simulink model "weightedSystem"  (R2015a)
settings: Solver=ode45  StartTime=0.0  StopTime=10.0  RelTol=1e-3
values from neighbouring files (symbols this model uses):
  Wz = ss(Wz)    [HinfSynthesis.m]
settings Model: Creator=anatole  LastModifiedBy=anatole

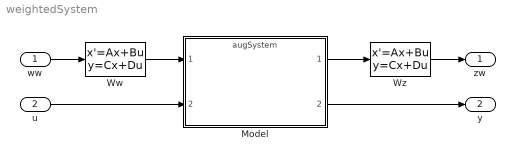
== system weightedSystem ==
  ww : Inport
  u : Inport  Port=2
  Model : ModelReference  ModelNameDialog=augSystem  SimulationMode=Normal  ModelReferenceVersion=1.3  CopyOfModelName=augSystem  DefaultDataLogging=on
  Ww : StateSpace  X0=0
  Wz : StateSpace  A=Wz.a  B=Wz.b  C=Wz.c  D=Wz.d  X0=0
  zw : Outport
  y : Outport  Port=2
  wires:
  Ww/1 -> Model/1
  Model/1 -> Wz/1
  ww/1 -> Ww/1
  Wz/1 -> zw/1
  Model/2 -> y/1
  u/1 -> Model/2
